simulink model "msd_04_Simulink_4"  (R2014a)
settings: Solver=ode45  StartTime=0.0  StopTime=10.0  MaxStep=0.01  RelTol=1e-3
InitFcn:
  | m = 3.600;     % kg
  | k = 400;    % N/m
  | b = 10;      % Ns/m
Description:
  | Copyright 2014 The MathWorks, Inc.
settings Model: Creator=smiller  LastModifiedBy=smiller
settings DebuggingCC: UnderspecifiedInitializationDetection=Classic  StateNameClashWarn=warning

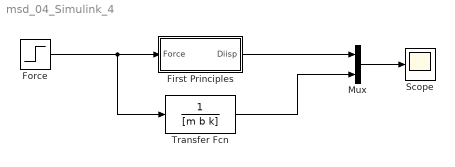
== system msd_04_Simulink_4 ==
  First Principles : Subsystem
  Force : Step  After=10  SampleTime=0
  Mux : Mux  Inputs=2
  Scope : Scope
  Transfer Fcn : TransferFcn  Denominator=[m b k]
  wires:
  Force/1 -> Transfer Fcn/1, First Principles/1(Force)
  First Principles/1(Diisp) -> Mux/1
  Mux/1 -> Scope/1
  Transfer Fcn/1 -> Mux/2

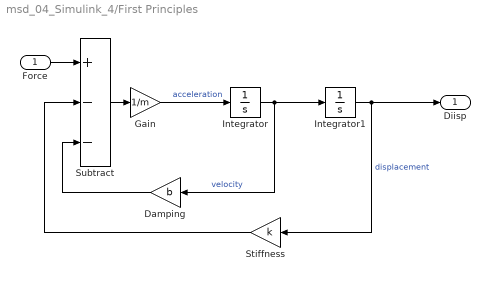
== system msd_04_Simulink_4/First Principles ==
  Force : Inport
  Damping : Gain  Gain=b
  Gain : Gain  Gain=1/m
  Integrator : Integrator
  Integrator1 : Integrator
  Stiffness : Gain  Gain=k
  Subtract : Sum  Inputs=+--
  Diisp : Outport
  wires:
  Force/1 -> Subtract/1
  Subtract/1 -> Gain/1
  Integrator/1 -> Damping/1, Integrator1/1  "velocity"
  Stiffness/1 -> Subtract/2
  Integrator1/1 -> Diisp/1, Stiffness/1  "displacement"
  Gain/1 -> Integrator/1  "acceleration"
  Damping/1 -> Subtract/3
